simulink model "parallel_8_delay_compensation"  (R2022a)
settings: Solver=FixedStepDiscrete  StartTime=0.0  StopTime=10.0  RelTol=1e-3
undefined symbols (not defined in the file or in its folder): f_c, L_d, L_q, L_x, L_y, p, psi_pm, R_ph
libraries: hdlsllib x2
settings Model: DataTypeOverride=Off  Creator=Andre Merx  LastModifiedBy=Andre Merx
settings SolverCC: AlgebraicLoopSolver=TrustRegion
settings DataIOCC: LimitDataPoints=on  SaveOutput=off  SaveTime=off
settings OptimizationCC: BlockReduction=off  ConditionallyExecuteInputs=off  DefaultParameterBehavior=Inlined  LifeSpan=inf
settings DebuggingCC: AlgebraicLoopMsg=error  SingleTaskRateTransMsg=error  UnconnectedInputMsg=warning  UnconnectedOutputMsg=warning  UnconnectedLineMsg=warning  AllowSymbolicDim=off  StrictBusMsg=ErrorOnBusTreatedAsVector  SFUnexpectedBacktrackingDiag=warning  SFNoUnconditionalDefaultTransitionDiag=warning  SFExecutionAtInitializationDiag=none  SFMachineParentedDataDiag=warning  ArithmeticOperatorsInVariantConditions=warning
settings HardwareCC: ProdBitPerPointer=32  ProdBitPerSizeT=32  ProdBitPerPtrDiffT=32  ProdLargestAtomicFloat=None  ProdIntDivRoundTo=Undefined  ProdEndianess=Unspecified  ProdWordSize=32  ProdHWDeviceType=ASIC/FPGA->ASIC/FPGA  ProdEqTarget=off
settings SFSimCC: SimUseLocalCustomCode=off  CustomCodeUndefinedFunction=UseInterfaceOnly
settings RTWCC: RTWUseLocalCustomCode=off
settings CodeAppCC: StateflowObjectComments=on
settings GRTTargetCC: TargetLangStandard=C89/C90 (ANSI)
settings ConfigComp: CovScope=ReferencedModels  CovMetricSettings=dw  CovSaveCumulativeToWorkspaceVar=on  CovSaveSingleToWorkspaceVar=on  CovExternalEMLEnable=off  CovSFcnEnable=off

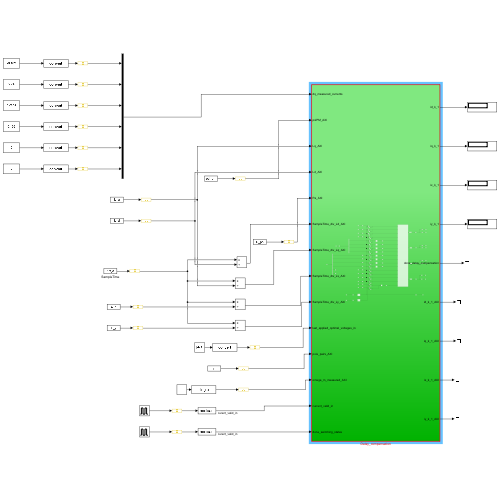
[thumbnail: Simulink's stored preview of the top-level diagram]
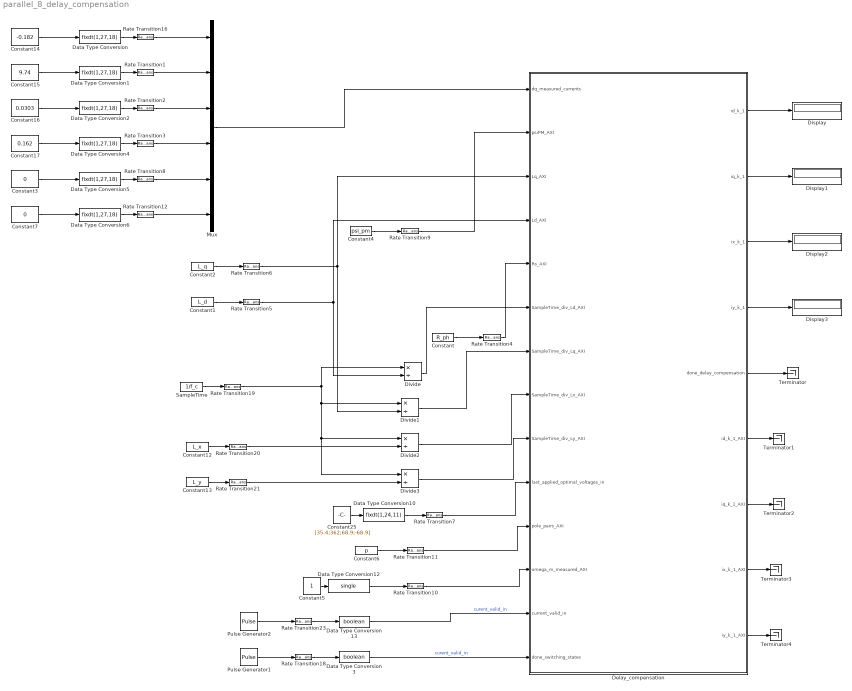
== system parallel_8_delay_compensation ==
  Constant : Constant  Value=R_ph  OutDataTypeStr=single  SampleTime=-1
  Constant1 : Constant  Value=L_d  OutDataTypeStr=single  SampleTime=-1
  Constant12 : Constant  Value=L_x  OutDataTypeStr=single  SampleTime=-1
  Constant13 : Constant  Value=L_y  OutDataTypeStr=single  SampleTime=-1
  Constant14 : Constant  Value=-0.182
  Constant15 : Constant  Value=9.74
  Constant16 : Constant  Value=0.0303
  Constant17 : Constant  Value=0.162
  Constant2 : Constant  Value=L_q  OutDataTypeStr=single  SampleTime=-1
  Constant25 : Constant  Value=[35.4;362;68.9;-68.9]
  Constant3 : Constant  Value=0
  Constant4 : Constant  Value=psi_pm  OutDataTypeStr=single  SampleTime=-1
  Constant5 : Constant
  Constant6 : Constant  Value=p  OutDataTypeStr=single  SampleTime=-1
  Constant7 : Constant  Value=0
  Data Type Conversion{,1..2,4..6} (6 alike) : DataTypeConversion  OutDataTypeStr=fixdt(1,27,18)  SaturateOnIntegerOverflow=off  RndMeth=Floor
  Data Type Conversion10 : DataTypeConversion  OutDataTypeStr=fixdt(1,24,11)  SaturateOnIntegerOverflow=off  RndMeth=Floor
  Data Type Conversion12 : DataTypeConversion  OutDataTypeStr=single  SaturateOnIntegerOverflow=off  RndMeth=Floor
  Data Type Conversion13 : DataTypeConversion  OutDataTypeStr=boolean  SaturateOnIntegerOverflow=off  RndMeth=Floor
  Data Type Conversion3 : DataTypeConversion  OutDataTypeStr=boolean  SaturateOnIntegerOverflow=off  RndMeth=Floor
  Delay_compensation : Subsystem  TreatAsAtomicUnit=on
  Display{,1..3} (4 alike) : Display
  Divide{,1..3} (4 alike) : Product  Inputs=*/  RndMeth=Zero  SaturateOnIntegerOverflow=on
  Mux : Mux  Inputs=6
  Pulse Generator1 : DiscretePulseGenerator  PulseType=Time based  Period=1/f_c
  Pulse Generator2 : DiscretePulseGenerator  PulseType=Time based  Period=1/f_c
  Rate Transition{1..12,16,18..21,23} (18 alike) : RateTransition  OutPortSampleTime=Rt
  SampleTime : Constant  Value=1/f_c  OutDataTypeStr=single  SampleTime=-1
  Terminator{,1..4} (5 alike) : Terminator
  wires:
  Rate Transition23/1 -> Data Type Conversion13/1
  Constant17/1 -> Data Type Conversion4/1
  Constant1/1 -> Rate Transition5/1
  Pulse Generator2/1 -> Rate Transition23/1
  Rate Transition19/1 -> Divide/1, Divide1/1, Divide3/1, Divide2/1
  Delay_compensation/5(done_delay_compensation) -> Terminator/1
  Pulse Generator1/1 -> Rate Transition18/1
  Delay_compensation/4(iy_k_1) -> Display3/1
  Delay_compensation/1(id_k_1) -> Display/1
  SampleTime/1 -> Rate Transition19/1
  Constant13/1 -> Rate Transition21/1
  Rate Transition4/1 -> Delay_compensation/5(Rs_AXI)
  Delay_compensation/3(ix_k_1) -> Display2/1
  Constant16/1 -> Data Type Conversion2/1
  Constant4/1 -> Rate Transition9/1
  Constant15/1 -> Data Type Conversion1/1
  Data Type Conversion2/1 -> Rate Transition2/1
  Data Type Conversion/1 -> Rate Transition16/1
  Data Type Conversion10/1 -> Rate Transition7/1
  Data Type Conversion1/1 -> Rate Transition1/1
  Delay_compensation/2(iq_k_1) -> Display1/1
  Rate Transition5/1 -> Delay_compensation/4(Ld_AXI), Divide/2
  Data Type Conversion4/1 -> Rate Transition3/1
  Data Type Conversion3/1 -> Delay_compensation/14(done_switching_states)  "curent_valid_in"
  Constant12/1 -> Rate Transition20/1
  Constant6/1 -> Rate Transition11/1
  Rate Transition18/1 -> Data Type Conversion3/1
  Divide3/1 -> Delay_compensation/9(SampleTime_div_Ly_AXI)
  Rate Transition10/1 -> Delay_compensation/12(omega_m_measured_AXI)
  Rate Transition21/1 -> Divide3/2
  Data Type Conversion12/1 -> Rate Transition10/1
  Data Type Conversion13/1 -> Delay_compensation/13(current_valid_in)  "curent_valid_in"
  Constant/1 -> Rate Transition4/1
  Divide2/1 -> Delay_compensation/8(SampleTime_div_Lx_AXI)
  Constant5/1 -> Data Type Conversion12/1
  Rate Transition7/1 -> Delay_compensation/10(last_applied_optimal_voltages_in)
  Rate Transition11/1 -> Delay_compensation/11(pole_pairs_AXI)
  Constant25/1 -> Data Type Conversion10/1
  Rate Transition20/1 -> Divide2/2
  Divide/1 -> Delay_compensation/6(SampleTime_div_Ld_AXI)
  Constant14/1 -> Data Type Conversion/1
  Divide1/1 -> Delay_compensation/7(SampleTime_div_Lq_AXI)
  Constant2/1 -> Rate Transition6/1
  Rate Transition9/1 -> Delay_compensation/2(psiPM_AXI)
  Rate Transition6/1 -> Delay_compensation/3(Lq_AXI), Divide1/2
  Delay_compensation/6(id_k_1_AXI) -> Terminator1/1
  Delay_compensation/7(iq_k_1_AXI) -> Terminator2/1
  Delay_compensation/8(ix_k_1_AXI) -> Terminator3/1
  Delay_compensation/9(iy_k_1_AXI) -> Terminator4/1
  Constant3/1 -> Data Type Conversion5/1
  Data Type Conversion5/1 -> Rate Transition8/1
  Constant7/1 -> Data Type Conversion6/1
  Data Type Conversion6/1 -> Rate Transition12/1
  Rate Transition8/1 -> Mux/5
  Rate Transition12/1 -> Mux/6
  Rate Transition16/1 -> Mux/1
  Rate Transition1/1 -> Mux/2
  Rate Transition2/1 -> Mux/3
  Rate Transition3/1 -> Mux/4
  Mux/1 -> Delay_compensation/1(dq_measured_currents)

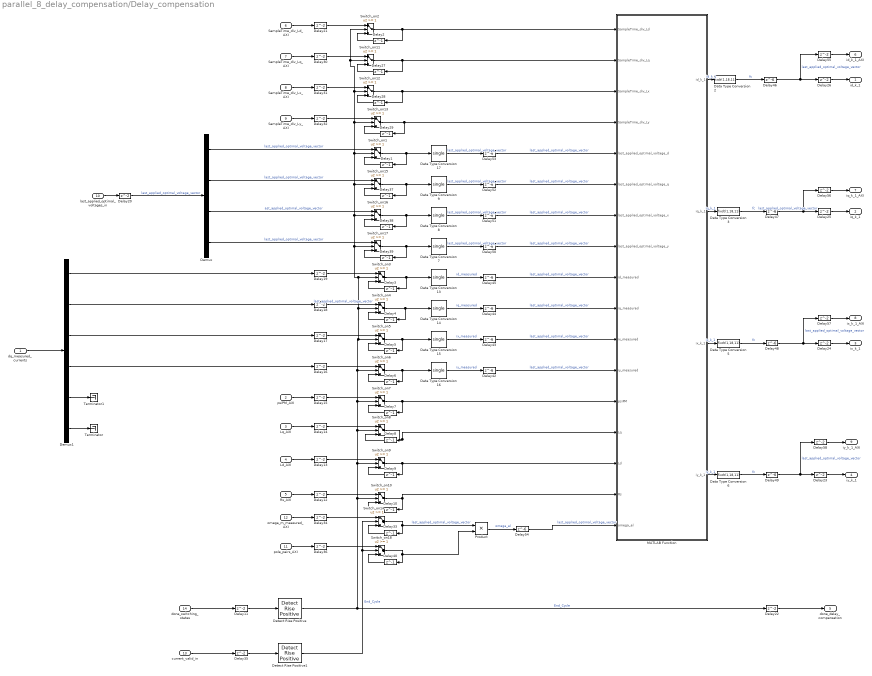
== system parallel_8_delay_compensation/Delay_compensation ==
  dq_measured_currents : Inport
  psiPM_AXI : Inport  Port=2
  Lq_AXI : Inport  Port=3
  Ld_AXI : Inport  Port=4
  Rs_AXI : Inport  Port=5
  SampleTime_div_Ld_AXI : Inport  Port=6
  SampleTime_div_Lq_AXI : Inport  Port=7
  SampleTime_div_Lx_AXI : Inport  Port=8
  SampleTime_div_Ly_AXI : Inport  Port=9
  last_applied_optimal_voltages_in : Inport  Port=10
  pole_pairs_AXI : Inport  Port=11
  omega_m_measured_AXI : Inport  Port=12
  current_valid_in : Inport  Port=13
  done_switching_states : Inport  Port=14
  Data Type Conversion{7..9,13..17} (8 alike) : DataTypeConversion  OutDataTypeStr=single  RndMeth=Nearest  SaturateOnIntegerOverflow=off
  Data Type Conversion{2..3,5..6} (4 alike) : DataTypeConversion  OutDataTypeStr=fixdt(1,18,11)  SaturateOnIntegerOverflow=off  RndMeth=Floor
  Delay{1..10,27..29,33,37..40} (18 alike) : Delay  DelayLength=1
  Delay{11..26,30..32,34..36,55..58} (26 alike) : Delay
  Delay{42..54} (13 alike) : Delay  DelayLength=6
  Demux : Demux
  Demux1 : Demux  Outputs=6
  Detect Rise Positive : hdlsllib/Logic and Bit Operations/Detect Rise Positive  vinit=0  OutDataTypeStr=boolean
      settings: SourceProductBaseCode=SL
  Detect Rise Positive1 : hdlsllib/Logic and Bit Operations/Detect Rise Positive  vinit=0  OutDataTypeStr=boolean
      settings: SourceProductBaseCode=SL
  MATLAB Function : MATLAB Function  TreatAsAtomicUnit=on  SystemSampleTime=1/100000000
  Product : Product  Inputs=**
  Switch_on{1..18} (18 alike) : Switch  Threshold=1  RndMeth=Simplest  SaturateOnIntegerOverflow=off  InputSameDT=off  OutDataTypeStr=Inherit: Same as first input
  Terminator : Terminator
  Terminator1 : Terminator
  id_k_1 : Outport
  iq_k_1 : Outport  Port=2
  ix_k_1 : Outport  Port=3
  iy_k_1 : Outport  Port=4
  done_delay_compensation : Outport  Port=5
  id_k_1_AXI : Outport  Port=6
  iq_k_1_AXI : Outport  Port=7
  ix_k_1_AXI : Outport  Port=8
  iy_k_1_AXI : Outport  Port=9
  wires:
  Delay33/1 -> Switch_on14/3
  pole_pairs_AXI/1 -> Delay36/1
  Delay9/1 -> Switch_on9/3
  Switch_on9/1 -> Delay9/1, MATLAB Function/15(Ld)
  Delay32/1 -> Switch_on13/1
  Lq_AXI/1 -> Delay14/1
  Delay31/1 -> Switch_on12/1
  Switch_on12/1 -> Delay28/1, MATLAB Function/3(SampleTime_div_Lx)
  Delay30/1 -> Switch_on11/1
  Delay29/1 -> Switch_on13/3
  SampleTime_div_Lx_AXI/1 -> Delay31/1
  Delay26/1 -> id_k_1/1
  Product/1 -> Delay54/1  "omega_el"
  Delay11/1 -> Detect Rise Positive/1
  Delay2/1 -> Switch_on2/3
  SampleTime_div_Lq_AXI/1 -> Delay30/1
  Switch_on5/1 -> Delay5/1, Data Type Conversion15/1
  Delay12/1 -> Switch_on10/1
  Rs_AXI/1 -> Delay12/1
  Delay1/1 -> Switch_on1/3
  Delay27/1 -> Switch_on11/3
  Delay21/1 -> Switch_on2/1
  Delay23/1 -> iy_k_1/1
  Delay24/1 -> ix_k_1/1
  Delay20/1 -> Demux/1  "last_applied_optimal_voltage_vector"
  Switch_on1/1 -> Delay1/1, Data Type Conversion17/1
  Delay8/1 -> Switch_on8/3
  Delay10/1 -> Switch_on10/3
  done_switching_states/1 -> Delay11/1
  Switch_on6/1 -> Delay6/1, Data Type Conversion16/1
  psiPM_AXI/1 -> Delay15/1
  Delay25/1 -> iq_k_1/1
  Switch_on13/1 -> Delay29/1, MATLAB Function/4(SampleTime_div_Ly)
  Switch_on4/1 -> Delay4/1, Data Type Conversion14/1
  Delay15/1 -> Switch_on7/1
  SampleTime_div_Ly_AXI/1 -> Delay32/1
  Switch_on10/1 -> Delay10/1, MATLAB Function/16(Rs)
  Delay7/1 -> Switch_on7/3
  Delay28/1 -> Switch_on12/3
  Switch_on8/1 -> Delay8/1, MATLAB Function/14(Lq)
  Ld_AXI/1 -> Delay13/1
  Delay6/1 -> Switch_on6/3
  Delay4/1 -> Switch_on4/3
  Switch_on11/1 -> Delay27/1, MATLAB Function/2(SampleTime_div_Lq)
  Delay3/1 -> Switch_on3/3
  Delay14/1 -> Switch_on8/1
  Switch_on2/1 -> Delay2/1, MATLAB Function/1(SampleTime_div_Ld)
  Delay22/1 -> done_delay_compensation/1
  Switch_on3/1 -> Delay3/1, Data Type Conversion13/1
  Delay13/1 -> Switch_on9/1
  Delay5/1 -> Switch_on5/3
  SampleTime_div_Ld_AXI/1 -> Delay21/1
  last_applied_optimal_voltages_in/1 -> Delay20/1
  omega_m_measured_AXI/1 -> Delay34/1
  Delay35/1 -> Detect Rise Positive1/1
  current_valid_in/1 -> Delay35/1
  Delay34/1 -> Switch_on14/1
  Delay36/1 -> Switch_on18/1
  Delay37/1 -> Switch_on15/3
  Delay38/1 -> Switch_on16/3
  Switch_on16/1 -> Data Type Conversion8/1, Delay38/1
  Delay39/1 -> Switch_on17/3
  Detect Rise Positive/1 -> Switch_on17/2, Switch_on16/2, Switch_on15/2, Switch_on13/2, Switch_on2/2, Switch_on11/2, Switch_on12/2, Switch_on1/2, Switch_on3/2, Switch_on4/2, Switch_on5/2, Switch_on6/2, Switch_on7/2, Switch_on8/2, Switch_on9/2, Switch_on10/2, Delay22/1  "End_Cycle"
  Switch_on17/1 -> Data Type Conversion7/1, Delay39/1
  Delay19/1 -> Switch_on3/1
  Delay18/1 -> Switch_on4/1  "last_applied_optimal_voltage_vector"
  Delay17/1 -> Switch_on5/1
  Delay16/1 -> Switch_on6/1
  MATLAB Function/1(id_k_1) -> Data Type Conversion2/1  "id_k_1"
  MATLAB Function/2(iq_k_1) -> Data Type Conversion3/1  "iq_k_1"
  MATLAB Function/3(ix_k_1) -> Data Type Conversion5/1  "ix_k_1"
  MATLAB Function/4(iy_k_1) -> Data Type Conversion6/1  "iy_k_1"
  Switch_on18/1 -> Product/2, Delay40/1
  Detect Rise Positive1/1 -> Switch_on18/2, Switch_on14/2  "End_Cycle"
  Delay40/1 -> Switch_on18/3
  Data Type Conversion13/1 -> Delay45/1  "id_measured"
  Data Type Conversion14/1 -> Delay44/1  "iq_measured"
  Data Type Conversion15/1 -> Delay43/1  "ix_measured"
  Data Type Conversion16/1 -> Delay42/1  "iy_measured"
  Switch_on7/1 -> MATLAB Function/13(psiPM), Delay7/1
  Switch_on15/1 -> Data Type Conversion9/1, Delay37/1
  Demux/1 -> Switch_on1/1  "last_applied_optimal_voltage_vector"
  Demux/2 -> Switch_on15/1  "last_applied_optimal_voltage_vector"
  Demux/3 -> Switch_on16/1  "ast_applied_optimal_voltage_vector"
  Demux/4 -> Switch_on17/1  "last_applied_optimal_voltage_vector"
  Data Type Conversion2/1 -> Delay46/1  "fc"
  Data Type Conversion3/1 -> Delay47/1  "fc"
  Data Type Conversion5/1 -> Delay48/1  "fc"
  Data Type Conversion6/1 -> Delay49/1  "fc"
  Switch_on14/1 -> Product/1, Delay33/1  "last_applied_optimal_voltage_vector"
  Delay42/1 -> MATLAB Function/12(iy_measured)  "last_applied_optimal_voltage_vector"
  Delay43/1 -> MATLAB Function/11(ix_measured)  "last_applied_optimal_voltage_vector"
  Delay44/1 -> MATLAB Function/10(iq_measured)  "last_applied_optimal_voltage_vector"
  Delay45/1 -> MATLAB Function/9(id_measured)  "last_applied_optimal_voltage_vector"
  Delay50/1 -> MATLAB Function/8(last_applied_optimal_voltage_y)  "last_applied_optimal_voltage_vector"
  Delay51/1 -> MATLAB Function/7(last_applied_optimal_voltage_x)  "last_applied_optimal_voltage_vector"
  Delay52/1 -> MATLAB Function/6(last_applied_optimal_voltage_q)  "last_applied_optimal_voltage_vector"
  Delay53/1 -> MATLAB Function/5(last_applied_optimal_voltage_d)  "last_applied_optimal_voltage_vector"
  Data Type Conversion7/1 -> Delay50/1  "last_applied_optimal_voltage_vector"
  Data Type Conversion8/1 -> Delay51/1  "last_applied_optimal_voltage_vector"
  Data Type Conversion9/1 -> Delay52/1  "last_applied_optimal_voltage_vector"
  Data Type Conversion17/1 -> Delay53/1  "last_applied_optimal_voltage_vector"
  Delay46/1 -> Delay55/1, Delay26/1  "last_applied_optimal_voltage_vector"
  Delay47/1 -> Delay56/1, Delay25/1  "last_applied_optimal_voltage_vector"
  Delay48/1 -> Delay57/1, Delay24/1  "last_applied_optimal_voltage_vector"
  Delay49/1 -> Delay58/1, Delay23/1  "last_applied_optimal_voltage_vector"
  Delay54/1 -> MATLAB Function/17(omega_el)  "last_applied_optimal_voltage_vector"
  Delay55/1 -> id_k_1_AXI/1
  Delay56/1 -> iq_k_1_AXI/1
  Delay57/1 -> ix_k_1_AXI/1
  Delay58/1 -> iy_k_1_AXI/1
  Demux1/2 -> Delay18/1
  Demux1/1 -> Delay19/1
  Demux1/4 -> Delay16/1
  Demux1/3 -> Delay17/1
  Demux1/6 -> Terminator/1
  Demux1/5 -> Terminator1/1
  dq_measured_currents/1 -> Demux1/1

== matlab function parallel_8_delay_compensation/Delay_compensation/MATLAB Function ==
  data: SampleTime_div_Ld input; SampleTime_div_Lq input; SampleTime_div_Lx input; SampleTime_div_Ly input; id_k_1 output; last_applied_optimal_voltage_d input; last_applied_optimal_voltage_q input; last_applied_optimal_voltage_x input; last_applied_optimal_voltage_y input; id_measured input; iq_measured input; ix_measured input; iy_measured input; psiPM input; Lq input; Ld input; Rs input; iq_k_1 output; ix_k_1 output; iy_k_1 output; omega_el input
function [id_k_1, iq_k_1, ix_k_1, iy_k_1] = fcn(SampleTime_div_Ld, SampleTime_div_Lq, SampleTime_div_Lx, SampleTime_div_Ly, last_applied_optimal_voltage_d, last_applied_optimal_voltage_q, last_applied_optimal_voltage_x, last_applied_optimal_voltage_y, id_measured, iq_measured, ix_measured, iy_measured, psiPM, Lq, Ld, Rs, omega_el)
  
    % Delay compensation with a modell of a 6-Phase PMSM
    id_k_1 = single(SampleTime_div_Ld*(last_applied_optimal_voltage_d-id_measured*Rs+omega_el*Lq*iq_measured)+id_measured);
    iq_k_1 = single(SampleTime_div_Lq*(last_applied_optimal_voltage_q-iq_measured*Rs-omega_el*(psiPM+id_measured*Ld))+iq_measured);
    ix_k_1 = single(SampleTime_div_Lx*(last_applied_optimal_voltage_x-ix_measured*Rs)+ix_measured);
    iy_k_1 = single(SampleTime_div_Ly*(last_applied_optimal_voltage_y-iy_measured*Rs)+iy_measured);

end
